simulink model "projectsimulink_20"  (R2023b)
settings: Solver=VariableStepAuto  StartTime=0.0  StopTime=10.0  MaxStep=1e-3  RelTol=1e-3
values from neighbouring files (symbols this model uses):
  g = 9.81    [Project_1.m]
  L = valuesOFlength(i)    [Project_1.m]
  theta0 = 10    [Project_1.m]

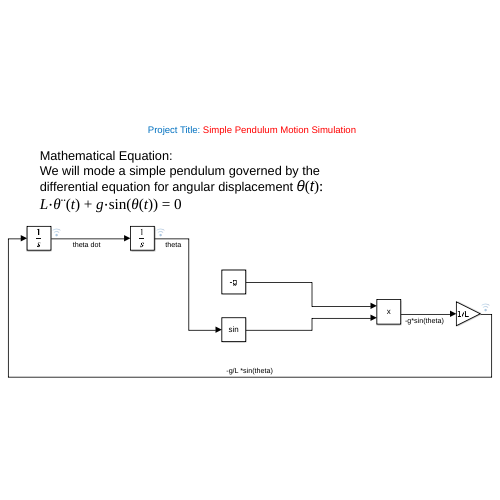
[thumbnail: Simulink's stored preview of the top-level diagram]
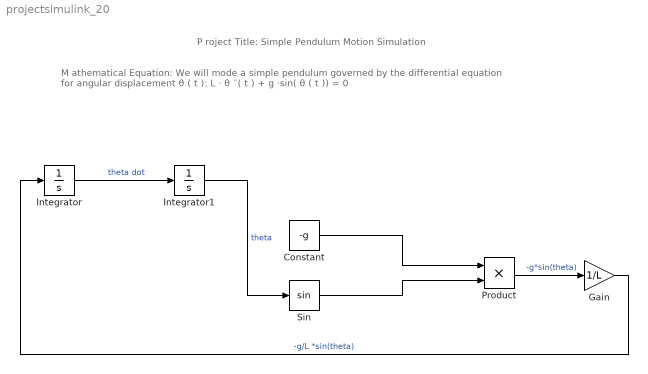
== system projectsimulink_20 ==
  note: P roject Title: Simple Pendulum Motion Simulation
  note: M athematical Equation:
      | We will mode a simple pendulum governed by the differential equation for angular displacement θ ( t ):
      | L ⋅ θ ¨( t ) + g ⋅sin( θ ( t )) = 0
  Constant : Constant  Value=-g
  Gain : Gain  Gain=1/L
  Integrator : Integrator
  Integrator1 : Integrator  InitialCondition=theta0
  Product : Product
  Sin : Trigonometry
  wires:
  Constant/1 -> Product/1
  Sin/1 -> Product/2
  Integrator1/1 -> Sin/1  "theta"
  Product/1 -> Gain/1  "-g*sin(theta)"
  Gain/1 -> Integrator/1  "-g/L *sin(theta)"
  Integrator/1 -> Integrator1/1  "theta dot"
